simulink model "multiple_msdft"  (R2013b)
settings: Solver=ode45  StartTime=0.0  StopTime=10.0  RelTol=1e-3
libraries: xbsIndex_r4 x13, sys_lib x6
settings Model: Creator=root  LastModifiedBy=root

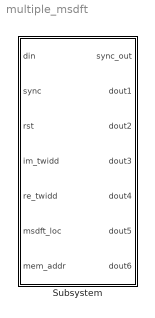
== system multiple_msdft ==
  Subsystem : Subsystem  mask{input_bitsize=8, fft_len=8, bin_range=[45 46 47 48 49 50], twid_bitsize=18, out_bitsize=20}
      mask prompts: input_bitsize "input bitsize"; fft_len "dft len (2^?)"; bin_range "bins"; twid_bitsize "twiddle bitsize"; out_bitsize "output bitsize"
      mask init:
      | config.source = str2func('msdft_init');
      | config.toplevel = gcb;
      | xBlock(config, {input_bitsize, fft_len, bin_range,...
      |             twid_bitsize, out_bitsize});

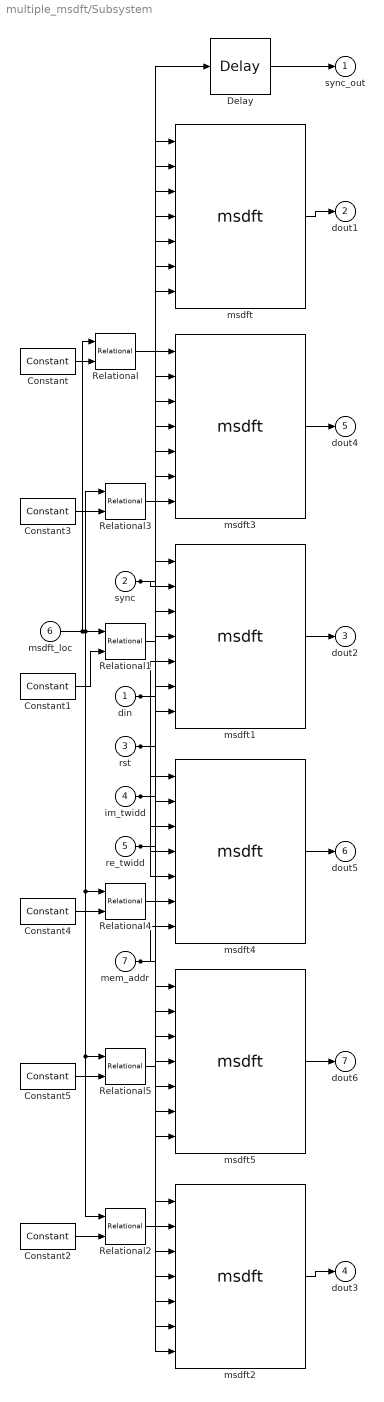
== system multiple_msdft/Subsystem ==
  din : Inport
  sync : Inport  Port=2
  rst : Inport  Port=3
  im_twidd : Inport  Port=4
  re_twidd : Inport  Port=5
  msdft_loc : Inport  Port=6
  mem_addr : Inport  Port=7
  Constant : xbsIndex_r4/Constant  const=0  gui_display_data_type=Fixed-point  arith_type=Unsigned  n_bits=10  bin_pt=0  preci_type=Single  exp_width=8  frac_width=24  explicit_period=on  period=1  equ=P=C  opselect=C  inp2=PCIN>>17  opr=+  inp1=P  carry=CIN  dbl_ovrd=off  block_type=constant
  Constant1 : xbsIndex_r4/Constant  const=1  gui_display_data_type=Fixed-point  arith_type=Unsigned  n_bits=10  bin_pt=0  preci_type=Single  exp_width=8  frac_width=24  explicit_period=on  period=1  equ=P=C  opselect=C  inp2=PCIN>>17  opr=+  inp1=P  carry=CIN  dbl_ovrd=off  block_type=constant
  Constant2 : xbsIndex_r4/Constant  const=2  gui_display_data_type=Fixed-point  arith_type=Unsigned  n_bits=10  bin_pt=0  preci_type=Single  exp_width=8  frac_width=24  explicit_period=on  period=1  equ=P=C  opselect=C  inp2=PCIN>>17  opr=+  inp1=P  carry=CIN  dbl_ovrd=off  block_type=constant
  Constant3 : xbsIndex_r4/Constant  const=3  gui_display_data_type=Fixed-point  arith_type=Unsigned  n_bits=10  bin_pt=0  preci_type=Single  exp_width=8  frac_width=24  explicit_period=on  period=1  equ=P=C  opselect=C  inp2=PCIN>>17  opr=+  inp1=P  carry=CIN  dbl_ovrd=off  block_type=constant
  Constant4 : xbsIndex_r4/Constant  const=4  gui_display_data_type=Fixed-point  arith_type=Unsigned  n_bits=10  bin_pt=0  preci_type=Single  exp_width=8  frac_width=24  explicit_period=on  period=1  equ=P=C  opselect=C  inp2=PCIN>>17  opr=+  inp1=P  carry=CIN  dbl_ovrd=off  block_type=constant
  Constant5 : xbsIndex_r4/Constant  const=5  gui_display_data_type=Fixed-point  arith_type=Unsigned  n_bits=10  bin_pt=0  preci_type=Single  exp_width=8  frac_width=24  explicit_period=on  period=1  equ=P=C  opselect=C  inp2=PCIN>>17  opr=+  inp1=P  carry=CIN  dbl_ovrd=off  block_type=constant
  Delay : xbsIndex_r4/Delay  rst=off  infoeditControl=Selection of Reset will increase slice count due to use of real FFs and instead of SRLs  en=off  latency=263  dbl_ovrd=off  reg_retiming=off  block_type=delay
  Relational{,1..5} (6 alike) : xbsIndex_r4/Relational  mode=a=b  en=off  latency=0  dbl_ovrd=off  block_type=relational
  msdft : sys_lib/msdft  in_bit=8  N=8  init_twidd=45  twidd_bit=18  out_bit=20
  msdft1 : sys_lib/msdft  in_bit=8  N=8  init_twidd=46  twidd_bit=18  out_bit=20
  msdft2 : sys_lib/msdft  in_bit=8  N=8  init_twidd=47  twidd_bit=18  out_bit=20
  msdft3 : sys_lib/msdft  in_bit=8  N=8  init_twidd=48  twidd_bit=18  out_bit=20
  msdft4 : sys_lib/msdft  in_bit=8  N=8  init_twidd=49  twidd_bit=18  out_bit=20
  msdft5 : sys_lib/msdft  in_bit=8  N=8  init_twidd=50  twidd_bit=18  out_bit=20
  sync_out : Outport
  dout1 : Outport  Port=2
  dout2 : Outport  Port=3
  dout3 : Outport  Port=4
  dout4 : Outport  Port=5
  dout5 : Outport  Port=6
  dout6 : Outport  Port=7
  wires:
  sync/1 -> msdft5/2, msdft4/2, msdft3/2, msdft2/2, msdft1/2, msdft/2, Delay/1
  msdft_loc/1 -> Relational5/1, Relational2/1, Relational4/1, Relational3/1, Relational1/1, Relational/1
  din/1 -> msdft5/1, msdft4/1, msdft3/1, msdft2/1, msdft1/1, msdft/1
  rst/1 -> msdft5/3, msdft4/3, msdft3/3, msdft2/3, msdft1/3, msdft/3
  im_twidd/1 -> msdft5/4, msdft4/4, msdft3/4, msdft2/4, msdft1/4, msdft/4
  re_twidd/1 -> msdft5/5, msdft4/5, msdft3/5, msdft2/5, msdft1/5, msdft/5
  mem_addr/1 -> msdft5/7, msdft4/7, msdft3/7, msdft2/7, msdft1/7, msdft/7
  msdft5/1 -> dout6/1
  Relational5/1 -> msdft5/6
  Constant5/1 -> Relational5/2
  msdft4/1 -> dout5/1
  Relational4/1 -> msdft4/6
  Constant4/1 -> Relational4/2
  msdft3/1 -> dout4/1
  Relational3/1 -> msdft3/6
  Constant3/1 -> Relational3/2
  msdft2/1 -> dout3/1
  Relational2/1 -> msdft2/6
  Constant2/1 -> Relational2/2
  msdft1/1 -> dout2/1
  Relational1/1 -> msdft1/6
  Constant1/1 -> Relational1/2
  msdft/1 -> dout1/1
  Relational/1 -> msdft/6
  Constant/1 -> Relational/2
  Delay/1 -> sync_out/1
